simulink model "closed_loop"  (R2023b)
settings: Solver=FixedStepAuto  StartTime=0.0  StopTime=10  FixedStep=1/1000  RelTol=1e-3  AbsTol=1e-3
model workspace: external: MATLAB File params.m (data not in the file)
values from neighbouring files (symbols this model uses):
  g = 9.81    [linearize_5states.m]
  m = 0.027    [linearize_5states.m]
libraries: nesl_utility x9
settings Model: Creator=Jocke  LastModifiedBy=75167
settings SolverCC: AutoScaleAbsTol=off  AlgebraicLoopSolver=TrustRegion
settings DataIOCC: ReturnWorkspaceOutputs=off
settings OptimizationCC: DefaultParameterBehavior=Inlined  UseDivisionForNetSlopeComputation=on  EnhancedBackFolding=on  PassReuseOutputArgsAs=Individual arguments  ZeroExternalMemoryAtStartup=off  ZeroInternalMemoryAtStartup=off  OptimizeBlockOrder=speed  DifferentSizesBufferReuse=on  OptimizationCustomize=off  EfficientTunableParamExpr=on
settings DebuggingCC: ParameterTunabilityLossMsg=error  UnconnectedInputMsg=warning  UnconnectedOutputMsg=warning  UnconnectedLineMsg=warning  ArithmeticOperatorsInVariantConditions=warning
settings ModelReferenceCC: EnableRefExpFcnMdlSchedulingChecks=on
settings SFSimCC: SimUseLocalCustomCode=off  MATLABDynamicMemAlloc=off  CustomCodeUndefinedFunction=UseInterfaceOnly
settings RTWCC: Description=Embedded Coder  SystemTargetFile=ert.tlc  TemplateMakefile=ert_default_tmf  RTWUseLocalCustomCode=off  Toolchain=GNU gcc/g++ | gmake (64-bit Linux)
settings CodeAppCC: ForceParamTrailComments=on  IgnoreCustomStorageClasses=off  OperatorAnnotations=on  SimulinkDataObjDesc=on  SFDataObjDesc=on  InsertBlockDesc=on
settings ERTTargetCC: TargetLangStandard=C99 (ISO)  GenerateSampleERTMain=on  InlinedParameterPlacement=NonHierarchical  ERTCustomFileTemplate=example_file_process.tlc
settings SimscapeCC: SimscapeNormalizeSystem=off  SimscapeLogType=all  SimscapeLogDataHistory=10000

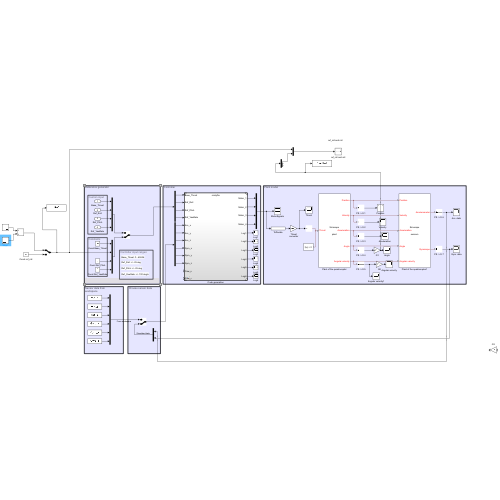
[thumbnail: Simulink's stored preview of the top-level diagram]
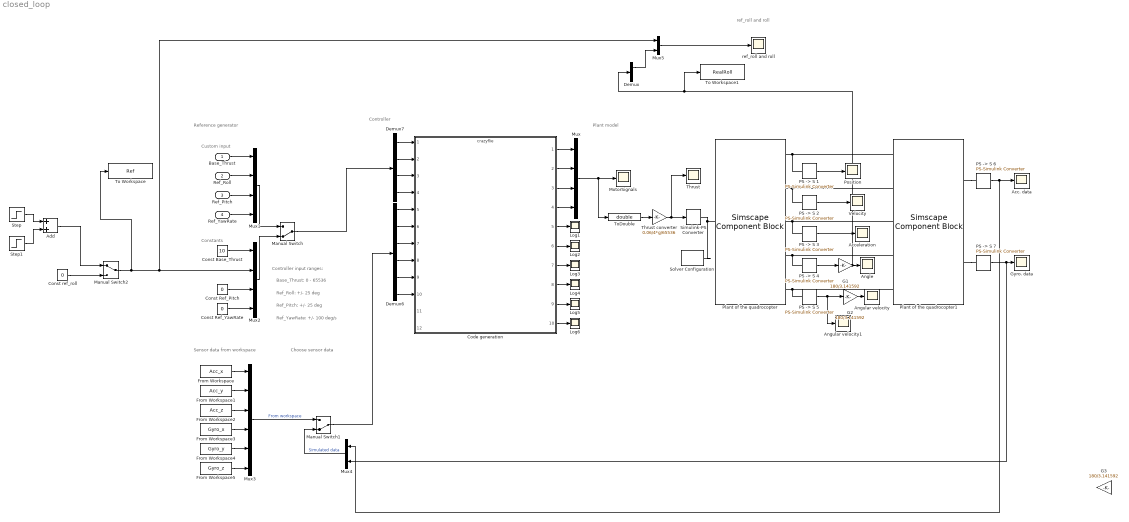
== system closed_loop ==
  note: ref_roll and roll
  note: Custom input
  note: Plant model
  note: Controller
  note: Constants
  note: Reference generator
  note: Ref_Roll: +/- 25 deg
  note: Base_Thrust: 0 - 65536
  note: Ref_Pitch: +/- 25 deg
  note: Ref_YawRate: +/- 100 deg/s
  note: Controller input ranges:
  note: Sensor data from
      | workspace
  note: Choose sensor data
  Base_Thrust : Inport  OutDataTypeStr=double
  Ref_Roll : Inport  Port=2  OutDataTypeStr=double
  Ref_Pitch : Inport  Port=3  OutDataTypeStr=double
  Ref_YawRate : Inport  Port=4  OutDataTypeStr=double
  Acc. data : Scope
  Acceleration : Scope
  Add : Sum
  Angle : Scope
  Angular velocity : Scope
  Angular velocity1 : Scope
  Code generation : ModelReference  ModelNameDialog=crazyflie.slx  SimulationMode=Normal  ModelReferenceVersion=9.8
  Const Base_Thrust : Constant  Value=10  SampleTime=0.01
  Const Ref_Pitch : Constant  Value=0  SampleTime=0.01
  Const Ref_YawRate : Constant  Value=0  SampleTime=0.01
  Const ref_roll : Constant  Value=0  SampleTime=0.01
  Demux : Demux  Outputs=3
  Demux6 : Demux  Outputs=6
  Demux7 : Demux
  From Workspace : FromWorkspace  VariableName=Acc_x  OutDataTypeStr=double
  From Workspace1 : FromWorkspace  VariableName=Acc_y  OutDataTypeStr=double
  From Workspace2 : FromWorkspace  VariableName=Acc_z  OutDataTypeStr=double
  From Workspace3 : FromWorkspace  VariableName=Gyro_x  OutDataTypeStr=double
  From Workspace4 : FromWorkspace  VariableName=Gyro_y  OutDataTypeStr=double
  From Workspace5 : FromWorkspace  VariableName=Gyro_z  OutDataTypeStr=double
  G1 : Gain  Gain=180/3.141592
  G2 : Gain  Gain=180/3.141592
  G3 : Gain  Gain=180/3.141592
  Gyro. data : Scope
  Log{1..6} (6 alike) : Scope
  Manual Switch : ManualSwitch  CurrentSetting=0
  Manual Switch1 : ManualSwitch  CurrentSetting=0
  Manual Switch2 : ManualSwitch
  MotorSignals : Scope
  Mux : Mux
  Mux1 : Mux
  Mux2 : Mux
  Mux3 : Mux  Inputs=6
  Mux4 : Mux  Inputs=2
  Mux5 : Mux  Inputs=2
  PS -> S {1..7} (7 alike) : nesl_utility/PS-Simulink Converter  PhysicalDomain=network_engine_domain  SubClassName=ps_output  LeftPortType=input  RightPortType=output  PseudoPeriodic=off  Frequencies=[]  VectorFormat=1-D array  Unit=1  AffineConversion=off
  Plant of the quadrocopter : SimscapeComponentBlock  SourceFile=plant  ComponentPath=plant  ComponentVariants=plant  ComponentVariantNames=plant  ClassName=plant  SchemaVersion=1  m=m kg  g=g m/s^2  d=d m  lift=lift N*s^2/rad^2  drag=drag N*m/(rad/s)^2  F=0.25 N*s/m
      settings: CopyFcn=simscape.engine.sli.internal.componentblockcallback(gcbh,'COPY')  PreCopyFcn=simscape.engine.sli.internal.componentblockcallback(gcbh,'PRECOPY')  PreDeleteFcn=simscape.engine.sli.internal.componentblockcallback(gcbh,'PREDELETE')  InternalSimscapePortConfiguration="{\"Bottom\":[],\"Left\":[{\"id\":\"ctrl\",\"label\":\"Thrust\",\"type\":\"input\"}],\"Right\":[{\"id\":\"pos\",\"label\":\"Position\",\"type\":\"output\"},{\"id\":\"v\",\"label\":\"Velocity\",\"type\":\"output\"},{\"id\":\"a\",\"label\":\"Acceleration\",\"type\":\"output\"},{\"id\":\"angle\",\"label\":\"Angle\",\"type\":\"output\"},{\"id\":\"w\",\"label\":\"Angular velocity\",\"type\":\"output\"}],\"Top\":[]}"
      mask Type: Plant of quadrocopter
  Plant of the quadrocopter1 : SimscapeComponentBlock  SourceFile=sensors  ComponentPath=sensors  ComponentVariants=sensors  ComponentVariantNames=sensors  ClassName=sensors  SchemaVersion=1  m=0.027 kg  g=9.81 m/s^2  d=0.046 m  k=2.5383e-11 m  b=1.9796e-9
      settings: CopyFcn=simscape.engine.sli.internal.componentblockcallback(gcbh,'COPY')  PreCopyFcn=simscape.engine.sli.internal.componentblockcallback(gcbh,'PRECOPY')  PreDeleteFcn=simscape.engine.sli.internal.componentblockcallback(gcbh,'PREDELETE')  InternalSimscapePortConfiguration="{\"Bottom\":[],\"Left\":[{\"id\":\"pos\",\"label\":\"Position\",\"type\":\"input\"},{\"id\":\"v\",\"label\":\"Velocity\",\"type\":\"input\"},{\"id\":\"a\",\"label\":\"Acceleration\",\"type\":\"input\"},{\"id\":\"angle\",\"label\":\"Angle\",\"type\":\"input\"},{\"id\":\"w\",\"label\":\"Angular velocity\",\"type\":\"input\"}],\"Right\":[{\"id\":\"acc\",\"label\":\"Accelerometer\",\"type\":\"output\"},{\"id\":\"gyro\",\"label\":\"Gyroscope\",\"type\":\"output\"}],\"Top\":[]}"
      mask Type: Plant of quadrocopter
  Position : Scope
  Simulink-PS Converter : nesl_utility/Simulink-PS Converter  PhysicalDomain=network_engine_domain  SubClassName=ps_input  LeftPortType=input  RightPortType=output  PseudoPeriodic=off  Frequencies=[]  NoiseDistribution=none  NoiseParameters=[]  Unit=1  AffineConversion=off  FilteringAndDerivatives=zero  SimscapeFilterOrder=1  InputFilterTimeConstant=0.001  UdotUserProvided=1
  Solver Configuration : nesl_utility/Solver Configuration  PhysicalDomain=network_engine_domain  SubClassName=solver  LeftPortType=input  RightPortType=generic  Tones=[]  Harmonics=[]  SimulateNoise=off  Profile=off  UseLocalSampling=off  EnableSwitchedLinearOptims=on  FrequencyDomain=off  UseCCode=off  RelTol=0.001  AbsTol=1e-06  MinStep=1e-09  ToWorkspace=off  RevertToSquareIcSolve=off  NumHomotopyIterations=100  PhasorMode=off  PhasorModeNumHarmonics=1  ConsistencySolver=NEWTON_FTOL  IndexReductionMethod=DerivativeReplacement  DoDC=off  ResidualTolerance=1e-09  ConsistencyTolSource=GLOBAL  ConsistencyAbsTol=0.001  ConsistencyRelTol=0.001  ConsistencyTolFactor=0.001  UseLocalSolver=off  LocalSolverChoice=NE_BACKWARD_EULER_ADVANCER  ResolveIndetEquations=on  FunctionEvalNumThread=1  LocalSolverSampleTime=0.001  DoFixedCost=off  MaxNonlinIter=3  MaxModeIter=2  ComputeImpulses=off  ImpulseIterations=2  LinearAlgebra=Sparse  LinearAlgebraNumThread=0  EquationFormulation=NE_TIME_EF  DelaysMemoryBudget=1024  AutomaticFiltering=on  FilteringTimeConstant=0.001  PartitionStorageMethod=AS_NEEDED  PartitionMemoryBudget=1024  PartitionMethod=FAST  MultibodyUseLocalSolver=off  MultibodyLocalSolverChoice=ODE1  MultibodyLocalSolverSampleTime=0.001
  Step : Step  Time=6.1  After=-6  SampleTime=0
  Step1 : Step  Time=6  After=6  SampleTime=0
  Thrust : Scope
  Thrust converter : Gain  Gain=0.06/4*g/65536
  To Workspace : ToWorkspace  VariableName=Ref  SaveFormat=Timeseries  SampleTime=-1
  To Workspace1 : ToWorkspace  VariableName=RealRoll  SaveFormat=Timeseries  SampleTime=-1
  ToDouble : DataTypeConversion  OutDataTypeStr=double  RndMeth=Round
  Velocity : Scope
  ref_roll and roll : Scope
  wires:
  Code generation/1 -> Mux/1
  Code generation/4 -> Mux/4
  Code generation/3 -> Mux/3
  Code generation/2 -> Mux/2
  "PS -> S 7"/1 -> Mux4/2, Gyro. data/1
  "PS -> S 6"/1 -> Mux4/1, Acc. data/1
  Code generation/5 -> Log1/1
  Code generation/6 -> Log2/1
  Code generation/7 -> Log3/1
  Code generation/8 -> Log4/1
  Code generation/9 -> Log5/1
  Code generation/10 -> Log6/1
  Mux/1 -> MotorSignals/1, ToDouble/1
  Base_Thrust/1 -> Mux1/1
  Ref_Roll/1 -> Mux1/2
  Ref_Pitch/1 -> Mux1/3
  Ref_YawRate/1 -> Mux1/4
  Mux1/1 -> Manual Switch/1
  Const Base_Thrust/1 -> Mux2/1
  Const Ref_Pitch/1 -> Mux2/3
  Const Ref_YawRate/1 -> Mux2/4
  Mux2/1 -> Manual Switch/2
  Manual Switch/1 -> Demux7/1
  Demux7/1 -> Code generation/1
  Demux7/2 -> Code generation/2
  Demux7/3 -> Code generation/3
  Demux7/4 -> Code generation/4
  G1/1 -> To Workspace1/1, Demux/1, Angle/1
  G2/1 -> Angular velocity/1
  ToDouble/1 -> Thrust converter/1
  Thrust converter/1 -> Thrust/1, Simulink-PS Converter/1
  "PS -> S 1"/1 -> Position/1
  "PS -> S 5"/1 -> Angular velocity1/1, G2/1
  "PS -> S 4"/1 -> G1/1
  "PS -> S 3"/1 -> Acceleration/1
  "PS -> S 2"/1 -> Velocity/1
  From Workspace5/1 -> Mux3/6
  From Workspace4/1 -> Mux3/5
  From Workspace3/1 -> Mux3/4
  From Workspace2/1 -> Mux3/3
  From Workspace1/1 -> Mux3/2
  From Workspace/1 -> Mux3/1
  Mux3/1 -> Manual Switch1/1  "From workspace"
  Demux6/1 -> Code generation/5
  Demux6/2 -> Code generation/6
  Demux6/3 -> Code generation/7
  Demux6/4 -> Code generation/8
  Demux6/5 -> Code generation/9
  Demux6/6 -> Code generation/10
  Manual Switch1/1 -> Demux6/1
  Mux4/1 -> Manual Switch1/2  "Simulated data"
  Mux5/1 -> ref_roll and roll/1
  Demux/1 -> Mux5/2
  Manual Switch2/1 -> To Workspace/1, Mux5/1, Mux2/2
  Const ref_roll/1 -> Manual Switch2/2
  Step/1 -> Add/1
  Step1/1 -> Add/2
  Add/1 -> Manual Switch2/1
  connections:
  Simulink-PS Converter/RConn1 -- Solver Configuration/RConn1 -- Plant of the quadrocopter/LConn1
  Plant of the quadrocopter1/LConn1 -- "PS -> S 1"/LConn1 -- Plant of the quadrocopter/RConn1
  Plant of the quadrocopter1/LConn2 -- "PS -> S 2"/LConn1 -- Plant of the quadrocopter/RConn2
  Plant of the quadrocopter1/LConn3 -- "PS -> S 3"/LConn1 -- Plant of the quadrocopter/RConn3
  Plant of the quadrocopter1/LConn4 -- "PS -> S 4"/LConn1 -- Plant of the quadrocopter/RConn4
  Plant of the quadrocopter1/LConn5 -- "PS -> S 5"/LConn1 -- Plant of the quadrocopter/RConn5
  Plant of the quadrocopter1/RConn1 -- "PS -> S 6"/LConn1
  Plant of the quadrocopter1/RConn2 -- "PS -> S 7"/LConn1
